simulink model "tempControlPI"  (R2013b)
settings: Solver=ode3  SolverMode=SingleTasking  StartTime=0.0  StopTime=800.0  RelTol=1e-3
libraries: arduino_io_lib x4
settings Model: ExtModeTrigDuration=2  Creator=gcampa  LastModifiedBy=Admin
settings OptimizationCC: OptimizeModelRefInitCode=on  LifeSpan=1
settings DebuggingCC: SolverPrmCheckMsg=none
settings HardwareCC: ProdBitPerInt=16  ProdBitPerPointer=8  ProdIntDivRoundTo=Zero  ProdEndianess=LittleEndian  ProdWordSize=8  ProdHWDeviceType=Atmel->AVR
settings RTWCC: SystemTargetFile=realtime.tlc  GenerateMakefile=off  TemplateMakefile=realtime.tmf  Description=Run on Target Hardware  RTWVerbose=off  ProcessScript=realtime_make_rtw_hook
settings STFCustomTargetCC: TargetLibSuffix=.a  GenerateSampleERTMain=on  ERTCustomFileBanners=on  SupportNonInlinedSFcns=off  SupportVariableSizeSignals=on  MATLABClassNameForMDSCustomization=Simulink.SoftwareTarget.ERTCustomization  GRTInterface=off  SystemTargetFile=realtime.tlc
settings ERTTargetCC: CodeReplacementLibrary=ANSI_C  GenerateSampleERTMain=on  ParMdlRefBuildCompliant=off  CompOptLevelCompliant=off  ConcurrentExecutionCompliant=off  CombineOutputUpdateFcns=off  ERTFirstTimeCompliant=off  SupportContinuousTime=on  SupportVariableSizeSignals=on  ModelStepFunctionPrototypeControlCompliant=off  CPPClassGenCompliant=off  ExtModeTransport=3  ExtModeMexFile=ext_serial_win32_comm  ExtModeMexArgs=0 1 9600  InlinedParameterPlacement=NonHierarchical  ERTSrcFileBannerTemplate=realtime_code_template.cgt  ERTHdrFileBannerTemplate=realtime_code_template.cgt  ERTDataSrcFileTemplate=realtime_code_template.cgt  ERTDataHdrFileTemplate=realtime_code_template.cgt  ERTCustomFileTemplate=realtime_file_process.tlc

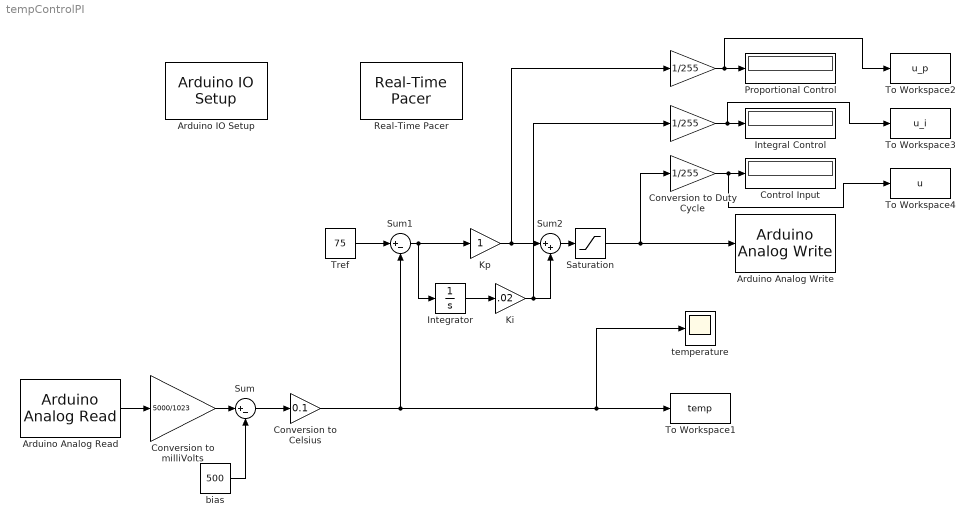
== system tempControlPI ==
  " " : Gain  Gain=1/255
  "  " : Gain  Gain=1/255
  Arduino Analog Read : arduino_io_lib/Arduino Analog Read  arduinoVar=Temporary arduino variable: Arduino1  arduinoPin=0  T=0.1
  Arduino Analog Write : arduino_io_lib/Arduino Analog Write  arduinoVar=Temporary arduino variable: Arduino1  arduinoPin=9  T=0.1
  Arduino IO Setup : arduino_io_lib/Arduino IO Setup  Priority=3  arduinoVar=Temporary arduino variable: Arduino1  workspaceVarName=b  comPort=COM3
  Control Input : Display
  Conversion to Celsius : Gain  Gain=0.1
  Conversion to Duty Cycle : Gain  Gain=1/255
  Conversion to milliVolts : Gain  Gain=5000/1023
  Integral Control : Display
  Integrator : Integrator
  Ki : Gain  Gain=.02
  Kp : Gain
  Proportional Control : Display
  Real-Time Pacer : arduino_io_lib/Real-Time Pacer  simTimePerRealTime=1
  Saturation : Saturate  UpperLimit=255  LowerLimit=0
  Sum : Sum  Inputs=|+-
  Sum1 : Sum  Inputs=|+-
  Sum2 : Sum  Inputs=|++
  To Workspace1 : ToWorkspace  VariableName=temp  SampleTime=-1  SaveFormat=Timeseries
  To Workspace2 : ToWorkspace  VariableName=u_p  SampleTime=-1  SaveFormat=Timeseries
  To Workspace3 : ToWorkspace  VariableName=u_i  SampleTime=-1  SaveFormat=Timeseries
  To Workspace4 : ToWorkspace  VariableName=u  SampleTime=-1  SaveFormat=Timeseries
  Tref : Constant  Value=75
  bias : Constant  Value=500
  temperature : Scope
      settings: YMin=15  YMax=120
  wires:
  Arduino Analog Read/1 -> Conversion to milliVolts/1
  Conversion to milliVolts/1 -> Sum/1
  Sum/1 -> Conversion to Celsius/1
  bias/1 -> Sum/2
  Tref/1 -> Sum1/1
  Conversion to Celsius/1 -> temperature/1, To Workspace1/1, Sum1/2
  Sum1/1 -> Integrator/1, Kp/1
  Saturation/1 -> Conversion to Duty Cycle/1, Arduino Analog Write/1
  Integrator/1 -> Ki/1
  Kp/1 -> "  "/1, Sum2/1
  Sum2/1 -> Saturation/1
  Ki/1 -> " "/1, Sum2/2
  Conversion to Duty Cycle/1 -> To Workspace4/1, Control Input/1
  " "/1 -> To Workspace3/1, Integral Control/1
  "  "/1 -> To Workspace2/1, Proportional Control/1
